simulink model "PMSM_SA88_1Motor"  (R2025a)
settings: Solver=ode4  StartTime=0.0  StopTime=StopTime  FixedStep=Ts_solver  RelTol=1e-3
values from neighbouring files (symbols this model uses):
  Bm = 1e-3    (= 0.001)    [EMRAX348_DQData.m]    (also in Evolito_D500_DQData.m; pmsm_batt_testbench_data.m)
  C1_pack = (Np/Ns)*c1_cell    [pmsm_batt_testbench_data.m]
  Cap_pack = Np*Cell_Cap    (= 700)    [pmsm_batt_testbench_data.m]
  Imax = 1070    [EMRAX348_DQData.m]    (also in Evolito_D500_DQData.m = 1450; pmsm_batt_testbench_data.m = 1450)
  Jtot = 2.0    (= 2)    [pmsm_batt_testbench_data.m]
  Ki_i = Rs*bw_i    (= 18.8495559215)    [pmsm_batt_testbench_data.m]
  Ki_w = Kp_w*bw_w/10    (= 292.432722995)    [pmsm_batt_testbench_data.m]
  Kp_i = Ld*bw_i    (= 0.251327412287)    [pmsm_batt_testbench_data.m]
  Kp_w = Jtot*bw_w/Kt    (= 93.084226773)    [pmsm_batt_testbench_data.m]
  Ld = 52e-6    (= 5.2e-05)    [EMRAX348_DQData.m]    (also in Evolito_D500_DQData.m = 4e-05; pmsm_batt_testbench_data.m = 4e-05)
  Lq = 52e-6    (= 5.2e-05)    [EMRAX348_DQData.m]    (also in Evolito_D500_DQData.m = 4e-05; pmsm_batt_testbench_data.m = 4e-05)
  OCV_pack = Ns*ocv_cell    [pmsm_batt_testbench_data.m]
  p = 10    [EMRAX348_DQData.m]    (also in Evolito_D500_DQData.m; pmsm_batt_testbench_data.m)
  psim = 0.06249    [EMRAX348_DQData.m]    (also in Evolito_D500_DQData.m = 0.045; pmsm_batt_testbench_data.m = 0.045)
  R0_pack = (Ns/Np)*rs_cell    [pmsm_batt_testbench_data.m]
  R1_pack = (Ns/Np)*r1_cell    [pmsm_batt_testbench_data.m]
  Rs = 0.00474    [EMRAX348_DQData.m]    (also in Evolito_D500_DQData.m = 0.004; pmsm_batt_testbench_data.m = 0.003)
  SOC0 = 0.90    (= 0.9)    [pmsm_batt_testbench_data.m]
  tau_dc = 1e-4    (= 0.0001)    [pmsm_batt_testbench_data.m]
  w_ref_val = [724.9; 726.5; 725.1; 726.7]    [pmsm_batt_testbench_data.m]
undefined symbols (not defined in the file or in its folder): soc_bp
libraries: slpidlib x3, simulink x1
settings Model: Creator=froshoo  LastModifiedBy=froshoo

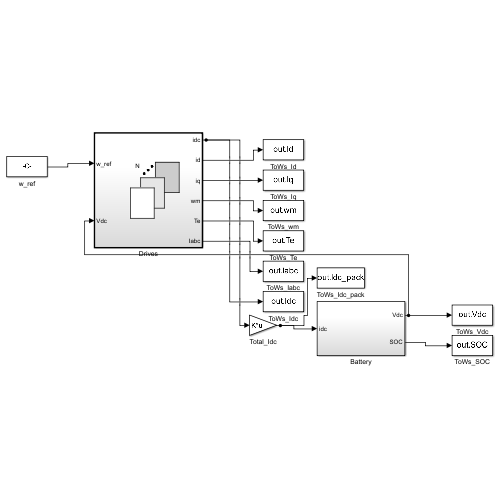
[thumbnail: Simulink's stored preview of the top-level diagram]
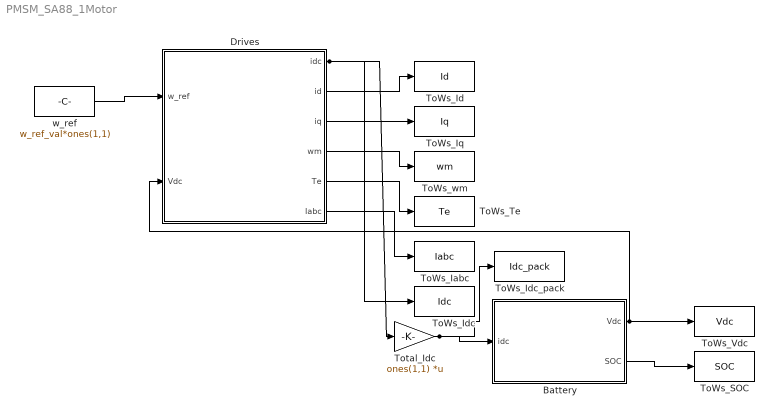
== system PMSM_SA88_1Motor ==
  Battery : Subsystem
  Drives : Subsystem  TreatAsAtomicUnit=on
  ToWs_Iabc : ToWorkspace  VariableName=Iabc  SaveFormat=Timeseries  SampleTime=-1
  ToWs_Id : ToWorkspace  VariableName=Id  SaveFormat=Timeseries  SampleTime=-1
  ToWs_Idc : ToWorkspace  VariableName=Idc  SaveFormat=Timeseries  SampleTime=-1
  ToWs_Idc_pack : ToWorkspace  VariableName=Idc_pack  SaveFormat=Timeseries  SampleTime=-1
  ToWs_Iq : ToWorkspace  VariableName=Iq  SaveFormat=Timeseries  SampleTime=-1
  ToWs_SOC : ToWorkspace  VariableName=SOC  SaveFormat=Timeseries  SampleTime=-1
  ToWs_Te : ToWorkspace  VariableName=Te  SaveFormat=Timeseries  SampleTime=-1
  ToWs_Vdc : ToWorkspace  VariableName=Vdc  SaveFormat=Timeseries  SampleTime=-1
  ToWs_wm : ToWorkspace  VariableName=wm  SaveFormat=Timeseries  SampleTime=-1
  Total_Idc : Gain  Gain=ones(1,1)  Multiplication=Matrix(K*u)
  w_ref : Constant  Value=w_ref_val*ones(1,1)
  wires:
  w_ref/1 -> Drives/1(w_ref)
  Battery/1(Vdc) -> Drives/2(Vdc), ToWs_Vdc/1
  Drives/1(idc) -> Total_Idc/1, ToWs_Idc/1
  Total_Idc/1 -> Battery/1(idc), ToWs_Idc_pack/1
  Drives/2(id) -> ToWs_Id/1
  Drives/3(iq) -> ToWs_Iq/1
  Drives/4(wm) -> ToWs_wm/1
  Drives/5(Te) -> ToWs_Te/1
  Drives/6(Iabc) -> ToWs_Iabc/1
  Battery/2(SOC) -> ToWs_SOC/1

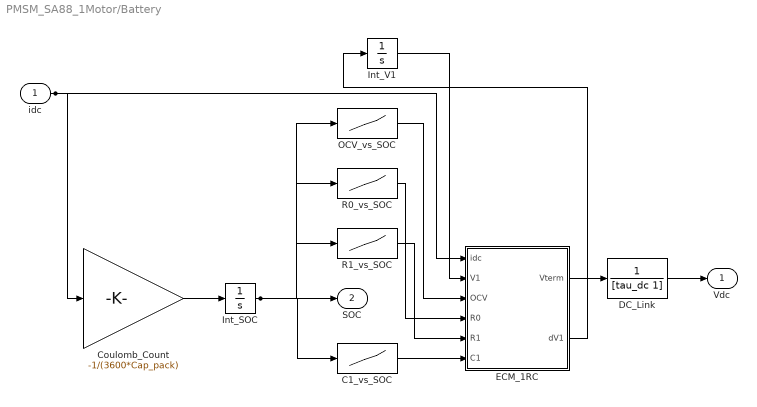
== system PMSM_SA88_1Motor/Battery ==
  idc : Inport
  C1_vs_SOC : Lookup_n-D  NumberOfTableDimensions=1  BreakpointsForDimension1=soc_bp  Table=C1_pack  InternalRulePriority=Speed  RndMeth=Simplest
  Coulomb_Count : Gain  Gain=-1/(3600*Cap_pack)
  DC_Link : TransferFcn  Denominator=[tau_dc 1]
  ECM_1RC : MATLAB Function  TreatAsAtomicUnit=on
  Int_SOC : Integrator  InitialCondition=SOC0
  Int_V1 : Integrator
  OCV_vs_SOC : Lookup_n-D  NumberOfTableDimensions=1  BreakpointsForDimension1=soc_bp  Table=OCV_pack  InternalRulePriority=Speed  RndMeth=Simplest
  R0_vs_SOC : Lookup_n-D  NumberOfTableDimensions=1  BreakpointsForDimension1=soc_bp  Table=R0_pack  InternalRulePriority=Speed  RndMeth=Simplest
  R1_vs_SOC : Lookup_n-D  NumberOfTableDimensions=1  BreakpointsForDimension1=soc_bp  Table=R1_pack  InternalRulePriority=Speed  RndMeth=Simplest
  Vdc : Outport
  SOC : Outport  Port=2
  wires:
  Int_V1/1 -> ECM_1RC/2(V1)
  idc/1 -> ECM_1RC/1(idc), Coulomb_Count/1
  Coulomb_Count/1 -> Int_SOC/1
  R0_vs_SOC/1 -> ECM_1RC/4(R0)
  Int_SOC/1 -> R0_vs_SOC/1, OCV_vs_SOC/1, SOC/1, C1_vs_SOC/1, R1_vs_SOC/1
  OCV_vs_SOC/1 -> ECM_1RC/3(OCV)
  R1_vs_SOC/1 -> ECM_1RC/5(R1)
  C1_vs_SOC/1 -> ECM_1RC/6(C1)
  ECM_1RC/2(dV1) -> Int_V1/1
  ECM_1RC/1(Vterm) -> DC_Link/1
  DC_Link/1 -> Vdc/1

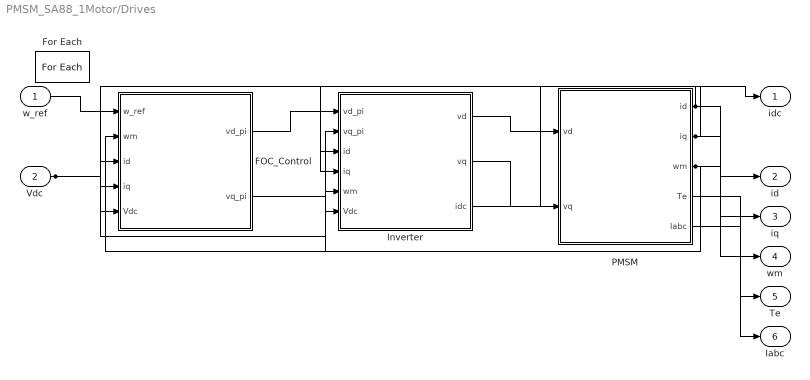
== system PMSM_SA88_1Motor/Drives ==
  w_ref : Inport  Partition=on  PartitionDimension=1  PartitionWidth=1  PartitionOffset=0
  Vdc : Inport  Port=2
  FOC_Control : Subsystem
  For Each : ForEach  DisableCoverage=on  SpecifiedNumIters=1
  Inverter : Subsystem
  PMSM : Subsystem
  idc : Outport  ConcatenationDimension=1
  id : Outport  Port=2  ConcatenationDimension=1
  iq : Outport  Port=3  ConcatenationDimension=1
  wm : Outport  Port=4  ConcatenationDimension=1
  Te : Outport  Port=5  ConcatenationDimension=1
  Iabc : Outport  Port=6  ConcatenationDimension=1
  wires:
  w_ref/1 -> FOC_Control/1(w_ref)
  PMSM/3(wm) -> FOC_Control/2(wm), Inverter/5(wm), wm/1
  PMSM/1(id) -> FOC_Control/3(id), Inverter/3(id), id/1
  PMSM/2(iq) -> FOC_Control/4(iq), Inverter/4(iq), iq/1
  Vdc/1 -> FOC_Control/5(Vdc), Inverter/6(Vdc)
  FOC_Control/1(vd_pi) -> Inverter/1(vd_pi)
  FOC_Control/2(vq_pi) -> Inverter/2(vq_pi)
  Inverter/1(vd) -> PMSM/1(vd)
  Inverter/2(vq) -> PMSM/2(vq)
  Inverter/3(idc) -> idc/1
  PMSM/4(Te) -> Te/1
  PMSM/5(Iabc) -> Iabc/1

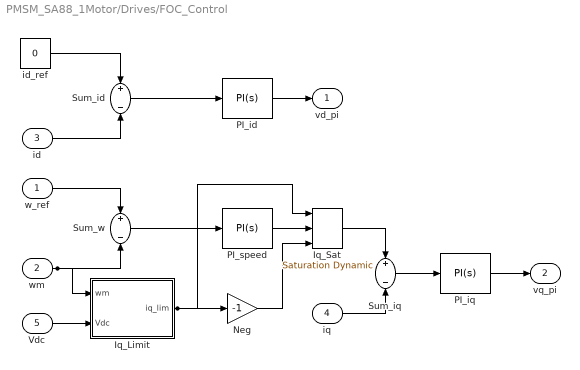
== system PMSM_SA88_1Motor/Drives/FOC_Control ==
  w_ref : Inport
  wm : Inport  Port=2
  id : Inport  Port=3
  iq : Inport  Port=4
  Vdc : Inport  Port=5
  Iq_Limit : MATLAB Function  TreatAsAtomicUnit=on
  Iq_Sat : simulink/Discontinuities/Saturation Dynamic  OutMin=[]  OutMax=[]  OutDataTypeStr=Inherit: Same as second input  OutDataType=fixdt(1, 16)  OutScaling=2^-10  DoSatur=off
  Neg : Gain  Gain=-1
  PI_id : slpidlib/PID Controller  Controller=PI  Form=Parallel  TimeDomain=Continuous-time  UseExternalTs=off  SampleTime=-1  IntegratorMethod=Forward Euler  FilterMethod=Forward Euler  ControllerParametersSource=internal  P=Kp_i  I=Ki_i  UseKiTs=off  D=0  UseExternalDerivativeSource=off  N=100  UseFilter=on  TunerSelectOption=Transfer Function Based (PID Tuner App)  InitialConditionSource=internal  InitialConditionForIntegrator=0  InitialConditionForFilter=0  DifferentiatorICPrevScaledInput=0  ExternalReset=none  TrackingMode=off  Kt=1  LimitOutput=off  SatLimitsSource=internal  UpperSaturationLimit=inf  LowerSaturationLimit=-inf  LinearizeAsGain=on  AntiWindupMode=none  Kb=1  LimitIntegrator=off  UpperIntegratorSaturationLimit=inf  LowerIntegratorSaturationLimit=-inf  POutMin=[]  POutMax=[]  IOutMin=[]  IOutMax=[]  DOutMin=[]  DOutMax=[]  NOutMin=[]  NOutMax=[]  SumOutMin=[]  SumOutMax=[]  SaturationOutMin=[]  SaturationOutMax=[]  PParamMin=[]  PParamMax=[]  IParamMin=[]  IParamMax=[]  DParamMin=[]  DParamMax=[]  NParamMin=[]  NParamMax=[]  KbParamMin=[]  KbParamMax=[]  KtParamMin=[]  KtParamMax=[]  KbOutMin=[]  KbOutMax=[]  KtOutMin=[]  KtOutMax=[]  IntegratorOutMin=[]  IntegratorOutMax=[]  FilterOutMin=[]  FilterOutMax=[]  SumI1OutMin=[]  SumI1OutMax=[]  SumI2OutMin=[]  SumI2OutMax=[]  SumI3OutMin=[]  SumI3OutMax=[]  SumI4OutMin=[]  SumI4OutMax=[]  SumDOutMin=[]  SumDOutMax=[]  DifferentiatorOutMin=[]  DifferentiatorOutMax=[]  FilterDiffOutCoefMin=[]  FilterDiffOutCoefMax=[]  ReciprocalOutMin=[]  ReciprocalOutMax=[]  SumDenOutMin=[]  SumDenOutMax=[]  SumNumOutMin=[]  SumNumOutMax=[]  DivideOutMin=[]  DivideOutMax=[]  UdiffTsProdOutMin=[]  UdiffTsProdOutMax=[]  NTsProdOutMin=[]  NTsProdOutMax=[]  UintegralTsProdOutMin=[]  UintegralTsProdOutMax=[]  UngainTsProdOutMin=[]  UngainTsProdOutMax=[]  ClampingZeroOutDataTypeStr=Inherit: Inherit via back propagation  ClampingZeroOutMin=[]  ClampingZeroOutMax=[]  FilterDenConstantOutDataTypeStr=Inherit: Inherit via back propagation  FilterDenConstantOutMin=[]  FilterDenConstantOutMax=[]  PCopyOutDataTypeStr=Inherit: Inherit via back propagation  PCopyOutMin=[]  PCopyOutMax=[]  NCopyOutDataTypeStr=Inherit: Inherit via back propagation  NCopyOutMin=[]  NCopyOutMax=[]  IntegratorContinuousStateAttributes=''  IntegratorStateMustResolveToSignalObject=off  IntegratorRTWStateStorageClass=Auto  FilterContinuousStateAttributes=''  FilterStateMustResolveToSignalObject=off  FilterRTWStateStorageClass=Auto  ParallelPVariant=InternalParameters  IdealPVariant=Disabled  IVariant=InternalParameters  DVariant=Disabled  IntegratorVariant=Continuous  SatVariant=Disabled  AWVariant=Passthrough  PCopyVariant=Disabled  TRVariant=Disabled  FdbkBlocksVariant=Forward  IdealPFdbkVariant=Disabled  SatFdbkVariant=Disabled  DerivativeFilterVariant=Disabled  NVariant=Disabled  NCopyVariant=Disabled_SignalSpec  FilterICVariant=Disabled  IntegratorICVariant=InternalICs  ExternalResetVariant=Disabled  TRSumVariant=Passthrough  SumFdbkVariant=Disabled  SumVariant=Sum_PI  TsampFilterVariant=InternalTs  TsampNgainVariant=Passthrough  TsampIntegralVariant=Disabled_SignalSpec  ExternalSaturationOutDataTypeStr=Inherit: Same as second input  DerivativeSourceVariant=Disabled  PreIntVariant=InternalPreInt
  PI_iq : slpidlib/PID Controller  Controller=PI  Form=Parallel  TimeDomain=Continuous-time  UseExternalTs=off  SampleTime=-1  IntegratorMethod=Forward Euler  FilterMethod=Forward Euler  ControllerParametersSource=internal  P=Kp_i  I=Ki_i  UseKiTs=off  D=0  UseExternalDerivativeSource=off  N=100  UseFilter=on  TunerSelectOption=Transfer Function Based (PID Tuner App)  InitialConditionSource=internal  InitialConditionForIntegrator=0  InitialConditionForFilter=0  DifferentiatorICPrevScaledInput=0  ExternalReset=none  TrackingMode=off  Kt=1  LimitOutput=off  SatLimitsSource=internal  UpperSaturationLimit=inf  LowerSaturationLimit=-inf  LinearizeAsGain=on  AntiWindupMode=none  Kb=1  LimitIntegrator=off  UpperIntegratorSaturationLimit=inf  LowerIntegratorSaturationLimit=-inf  POutMin=[]  POutMax=[]  IOutMin=[]  IOutMax=[]  DOutMin=[]  DOutMax=[]  NOutMin=[]  NOutMax=[]  SumOutMin=[]  SumOutMax=[]  SaturationOutMin=[]  SaturationOutMax=[]  PParamMin=[]  PParamMax=[]  IParamMin=[]  IParamMax=[]  DParamMin=[]  DParamMax=[]  NParamMin=[]  NParamMax=[]  KbParamMin=[]  KbParamMax=[]  KtParamMin=[]  KtParamMax=[]  KbOutMin=[]  KbOutMax=[]  KtOutMin=[]  KtOutMax=[]  IntegratorOutMin=[]  IntegratorOutMax=[]  FilterOutMin=[]  FilterOutMax=[]  SumI1OutMin=[]  SumI1OutMax=[]  SumI2OutMin=[]  SumI2OutMax=[]  SumI3OutMin=[]  SumI3OutMax=[]  SumI4OutMin=[]  SumI4OutMax=[]  SumDOutMin=[]  SumDOutMax=[]  DifferentiatorOutMin=[]  DifferentiatorOutMax=[]  FilterDiffOutCoefMin=[]  FilterDiffOutCoefMax=[]  ReciprocalOutMin=[]  ReciprocalOutMax=[]  SumDenOutMin=[]  SumDenOutMax=[]  SumNumOutMin=[]  SumNumOutMax=[]  DivideOutMin=[]  DivideOutMax=[]  UdiffTsProdOutMin=[]  UdiffTsProdOutMax=[]  NTsProdOutMin=[]  NTsProdOutMax=[]  UintegralTsProdOutMin=[]  UintegralTsProdOutMax=[]  UngainTsProdOutMin=[]  UngainTsProdOutMax=[]  ClampingZeroOutDataTypeStr=Inherit: Inherit via back propagation  ClampingZeroOutMin=[]  ClampingZeroOutMax=[]  FilterDenConstantOutDataTypeStr=Inherit: Inherit via back propagation  FilterDenConstantOutMin=[]  FilterDenConstantOutMax=[]  PCopyOutDataTypeStr=Inherit: Inherit via back propagation  PCopyOutMin=[]  PCopyOutMax=[]  NCopyOutDataTypeStr=Inherit: Inherit via back propagation  NCopyOutMin=[]  NCopyOutMax=[]  IntegratorContinuousStateAttributes=''  IntegratorStateMustResolveToSignalObject=off  IntegratorRTWStateStorageClass=Auto  FilterContinuousStateAttributes=''  FilterStateMustResolveToSignalObject=off  FilterRTWStateStorageClass=Auto  ParallelPVariant=InternalParameters  IdealPVariant=Disabled  IVariant=InternalParameters  DVariant=Disabled  IntegratorVariant=Continuous  SatVariant=Disabled  AWVariant=Passthrough  PCopyVariant=Disabled  TRVariant=Disabled  FdbkBlocksVariant=Forward  IdealPFdbkVariant=Disabled  SatFdbkVariant=Disabled  DerivativeFilterVariant=Disabled  NVariant=Disabled  NCopyVariant=Disabled_SignalSpec  FilterICVariant=Disabled  IntegratorICVariant=InternalICs  ExternalResetVariant=Disabled  TRSumVariant=Passthrough  SumFdbkVariant=Disabled  SumVariant=Sum_PI  TsampFilterVariant=InternalTs  TsampNgainVariant=Passthrough  TsampIntegralVariant=Disabled_SignalSpec  ExternalSaturationOutDataTypeStr=Inherit: Same as second input  DerivativeSourceVariant=Disabled  PreIntVariant=InternalPreInt
  PI_speed : slpidlib/PID Controller  Controller=PI  Form=Parallel  TimeDomain=Continuous-time  UseExternalTs=off  SampleTime=-1  IntegratorMethod=Forward Euler  FilterMethod=Forward Euler  ControllerParametersSource=internal  P=Kp_w  I=Ki_w  UseKiTs=off  D=0  UseExternalDerivativeSource=off  N=100  UseFilter=on  TunerSelectOption=Transfer Function Based (PID Tuner App)  InitialConditionSource=internal  InitialConditionForIntegrator=0  InitialConditionForFilter=0  DifferentiatorICPrevScaledInput=0  ExternalReset=none  TrackingMode=off  Kt=1  LimitOutput=on  SatLimitsSource=internal  UpperSaturationLimit=Imax  LowerSaturationLimit=-Imax  LinearizeAsGain=on  AntiWindupMode=back-calculation  Kb=1  LimitIntegrator=off  UpperIntegratorSaturationLimit=inf  LowerIntegratorSaturationLimit=-inf  POutMin=[]  POutMax=[]  IOutMin=[]  IOutMax=[]  DOutMin=[]  DOutMax=[]  NOutMin=[]  NOutMax=[]  SumOutMin=[]  SumOutMax=[]  SaturationOutMin=[]  SaturationOutMax=[]  PParamMin=[]  PParamMax=[]  IParamMin=[]  IParamMax=[]  DParamMin=[]  DParamMax=[]  NParamMin=[]  NParamMax=[]  KbParamMin=[]  KbParamMax=[]  KtParamMin=[]  KtParamMax=[]  KbOutMin=[]  KbOutMax=[]  KtOutMin=[]  KtOutMax=[]  IntegratorOutMin=[]  IntegratorOutMax=[]  FilterOutMin=[]  FilterOutMax=[]  SumI1OutMin=[]  SumI1OutMax=[]  SumI2OutMin=[]  SumI2OutMax=[]  SumI3OutMin=[]  SumI3OutMax=[]  SumI4OutMin=[]  SumI4OutMax=[]  SumDOutMin=[]  SumDOutMax=[]  DifferentiatorOutMin=[]  DifferentiatorOutMax=[]  FilterDiffOutCoefMin=[]  FilterDiffOutCoefMax=[]  ReciprocalOutMin=[]  ReciprocalOutMax=[]  SumDenOutMin=[]  SumDenOutMax=[]  SumNumOutMin=[]  SumNumOutMax=[]  DivideOutMin=[]  DivideOutMax=[]  UdiffTsProdOutMin=[]  UdiffTsProdOutMax=[]  NTsProdOutMin=[]  NTsProdOutMax=[]  UintegralTsProdOutMin=[]  UintegralTsProdOutMax=[]  UngainTsProdOutMin=[]  UngainTsProdOutMax=[]  ClampingZeroOutDataTypeStr=Inherit: Inherit via back propagation  ClampingZeroOutMin=[]  ClampingZeroOutMax=[]  FilterDenConstantOutDataTypeStr=Inherit: Inherit via back propagation  FilterDenConstantOutMin=[]  FilterDenConstantOutMax=[]  PCopyOutDataTypeStr=Inherit: Inherit via back propagation  PCopyOutMin=[]  PCopyOutMax=[]  NCopyOutDataTypeStr=Inherit: Inherit via back propagation  NCopyOutMin=[]  NCopyOutMax=[]  IntegratorContinuousStateAttributes=''  IntegratorStateMustResolveToSignalObject=off  IntegratorRTWStateStorageClass=Auto  FilterContinuousStateAttributes=''  FilterStateMustResolveToSignalObject=off  FilterRTWStateStorageClass=Auto  ParallelPVariant=InternalParameters  IdealPVariant=Disabled  IVariant=InternalParameters  DVariant=Disabled  IntegratorVariant=Continuous  SatVariant=Enabled  AWVariant=BackCalculation  PCopyVariant=Disabled  TRVariant=Disabled  FdbkBlocksVariant=Forward  IdealPFdbkVariant=Disabled  SatFdbkVariant=Disabled  DerivativeFilterVariant=Disabled  NVariant=Disabled  NCopyVariant=Disabled_SignalSpec  FilterICVariant=Disabled  IntegratorICVariant=InternalICs  ExternalResetVariant=Disabled  TRSumVariant=Passthrough  SumFdbkVariant=Disabled  SumVariant=Sum_PI  TsampFilterVariant=InternalTs  TsampNgainVariant=Passthrough  TsampIntegralVariant=Disabled_SignalSpec  ExternalSaturationOutDataTypeStr=Inherit: Same as second input  DerivativeSourceVariant=Disabled  PreIntVariant=InternalPreInt
  Sum_id : Sum  Inputs=+-
  Sum_iq : Sum  Inputs=+-
  Sum_w : Sum  Inputs=+-
  id_ref : Constant  Value=0
  vd_pi : Outport
  vq_pi : Outport  Port=2
  wires:
  Vdc/1 -> Iq_Limit/2(Vdc)
  id_ref/1 -> Sum_id/1
  wm/1 -> Sum_w/2, Iq_Limit/1(wm)
  PI_iq/1 -> vq_pi/1
  w_ref/1 -> Sum_w/1
  id/1 -> Sum_id/2
  Sum_iq/1 -> PI_iq/1
  Sum_id/1 -> PI_id/1
  Sum_w/1 -> PI_speed/1
  Iq_Limit/1(iq_lim) -> Iq_Sat/1, Neg/1
  PI_id/1 -> vd_pi/1
  PI_speed/1 -> Iq_Sat/2
  Neg/1 -> Iq_Sat/3
  Iq_Sat/1 -> Sum_iq/1
  iq/1 -> Sum_iq/2

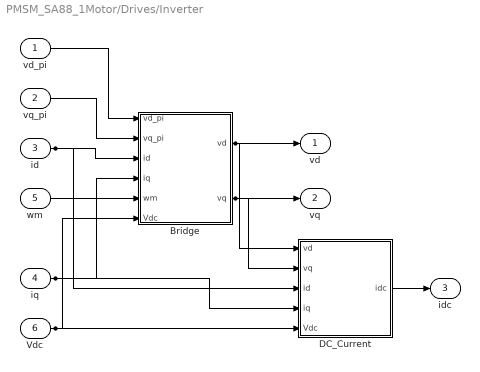
== system PMSM_SA88_1Motor/Drives/Inverter ==
  vd_pi : Inport
  vq_pi : Inport  Port=2
  id : Inport  Port=3
  iq : Inport  Port=4
  wm : Inport  Port=5
  Vdc : Inport  Port=6
  Bridge : MATLAB Function  TreatAsAtomicUnit=on
  DC_Current : MATLAB Function  TreatAsAtomicUnit=on
  vd : Outport
  vq : Outport  Port=2
  idc : Outport  Port=3
  wires:
  vd_pi/1 -> Bridge/1(vd_pi)
  vq_pi/1 -> Bridge/2(vq_pi)
  Vdc/1 -> DC_Current/5(Vdc), Bridge/6(Vdc)
  id/1 -> DC_Current/3(id), Bridge/3(id)
  Bridge/1(vd) -> vd/1, DC_Current/1(vd)
  wm/1 -> Bridge/5(wm)
  Bridge/2(vq) -> vq/1, DC_Current/2(vq)
  iq/1 -> Bridge/4(iq), DC_Current/4(iq)
  DC_Current/1(idc) -> idc/1

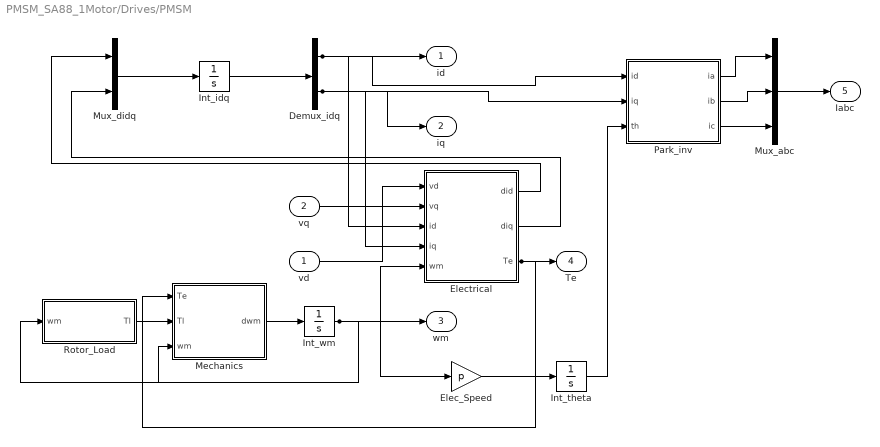
== system PMSM_SA88_1Motor/Drives/PMSM ==
  vd : Inport
  vq : Inport  Port=2
  Demux_idq : Demux  Outputs=2
  Elec_Speed : Gain  Gain=p
  Electrical : MATLAB Function  TreatAsAtomicUnit=on
  Int_idq : Integrator  InitialCondition=[0;0]
  Int_theta : Integrator
  Int_wm : Integrator
  Mechanics : MATLAB Function  TreatAsAtomicUnit=on
  Mux_abc : Mux  Inputs=3
  Mux_didq : Mux  Inputs=2
  Park_inv : MATLAB Function  TreatAsAtomicUnit=on
  Rotor_Load : MATLAB Function  TreatAsAtomicUnit=on
  id : Outport
  iq : Outport  Port=2
  wm : Outport  Port=3
  Te : Outport  Port=4
  Iabc : Outport  Port=5
  wires:
  Mux_didq/1 -> Int_idq/1
  Demux_idq/2 -> Park_inv/2(iq), Electrical/4(iq), iq/1
  Rotor_Load/1(Tl) -> Mechanics/2(Tl)
  Mux_abc/1 -> Iabc/1
  Park_inv/2(ib) -> Mux_abc/2
  vd/1 -> Electrical/1(vd)
  Int_idq/1 -> Demux_idq/1
  Mechanics/1(dwm) -> Int_wm/1
  Demux_idq/1 -> Park_inv/1(id), Electrical/3(id), id/1
  vq/1 -> Electrical/2(vq)
  Int_wm/1 -> Rotor_Load/1(wm), Electrical/5(wm), wm/1, Mechanics/3(wm), Elec_Speed/1
  Electrical/3(Te) -> Mechanics/1(Te), Te/1
  Electrical/1(did) -> Mux_didq/1
  Electrical/2(diq) -> Mux_didq/2
  Elec_Speed/1 -> Int_theta/1
  Int_theta/1 -> Park_inv/3(th)
  Park_inv/1(ia) -> Mux_abc/1
  Park_inv/3(ic) -> Mux_abc/3

== matlab function PMSM_SA88_1Motor/Battery/ECM_1RC ==
  data: idc input size=1; Vterm output size=1; V1 input size=1; OCV input size=1; R0 input size=1; R1 input size=1; C1 input size=1; dV1 output size=1
function [Vterm, dV1] = fcn(idc, V1, OCV, R0, R1, C1)
%#codegen
% SA88 pack, 1-RC equivalent-circuit model. idc is the TOTAL pack current
% (all motors summed). Discharge (idc > 0) pulls the terminal voltage below
% the open-circuit voltage -- this is what couples the motors to each other.
%   Vterm = OCV(SOC) - idc*R0(SOC) - V1
%   dV1/dt = idc/C1 - V1/(R1*C1)
Vterm = OCV - idc*R0 - V1;
dV1   = idc/C1 - V1/(R1*C1);

== matlab function PMSM_SA88_1Motor/Drives/Inverter/Bridge ==
  data: vd_pi input size=1; vd output size=1; vq_pi input size=1; id input size=1; iq input size=1; wm input size=1; Vdc input size=1; vq output size=1; p parameter; Ld parameter; Lq parameter; psim parameter
function [vd, vq] = fcn(vd_pi, vq_pi, id, iq, wm, Vdc, p, Ld, Lq, psim)
%#codegen
% Averaged inverter: no switching, so no PWM ripple -- the dq voltage command
% is applied directly. Two things happen here:
%  1) dq decoupling feedforward. The PI outputs only have to cover the
%     resistive drop and transients; the back-EMF and the we*L cross-coupling
%     are cancelled. Without this the d-axis loses control near the voltage
%     limit and id drifts positive (which raises the flux and makes it worse).
%  2) clamp onto the SVPWM linear-range circle, Vmax = Vdc/sqrt(3).
we   = p*wm;
vd_c = vd_pi - we*Lq*iq;
vq_c = vq_pi + we*(Ld*id + psim);
Vmax = Vdc/sqrt(3);
Vm   = sqrt(vd_c^2 + vq_c^2);
if Vm > Vmax && Vm > 0
    k = Vmax/Vm;
else
    k = 1;
end
vd = k*vd_c;
vq = k*vq_c;

== matlab function PMSM_SA88_1Motor/Drives/FOC_Control/Iq_Limit ==
  data: wm input size=1; iq_lim output size=1; Vdc input size=1; p parameter; psim parameter; Lq parameter; Imax parameter
function iq_lim = fcn(wm, Vdc, p, psim, Lq, Imax)
%#codegen
% Largest iq the bus can actually drive at this speed (with id = 0):
%   (we*psim + Rs*iq)^2 + (we*Lq*iq)^2 <= Vmax^2
% Dropping the small Rs*iq term -> iq <= sqrt(Vmax^2-(we*psim)^2)/(we*Lq).
% A flat Imax limit would command an iq the bus cannot support, the inverter
% would saturate and the current PIs would wind up (id runs away).
we   = p*abs(wm);
Vmax = Vdc/sqrt(3);
Eb   = we*psim;
marg = Vmax^2 - Eb^2;
if we < 1 || marg <= 0
    iq_v = Imax;
else
    iq_v = sqrt(marg)/(we*Lq);
end
iq_lim = min(Imax, iq_v);

== matlab function PMSM_SA88_1Motor/Drives/Inverter/DC_Current ==
  data: vd input size=1; idc output size=1; vq input size=1; id input size=1; iq input size=1; Vdc input size=1
function idc = fcn(vd, vq, id, iq, Vdc)
%#codegen
% DC-side current from AC power balance (averaged inverter, lossless).
% This is what ties the AC side to the battery: Pdc = Pac.
Pac = 1.5*(vd*id + vq*iq);
idc = Pac/max(Vdc, 1);

== matlab function PMSM_SA88_1Motor/Drives/PMSM/Electrical ==
  data: vd input size=1; did output size=1; vq input size=1; id input size=1; iq input size=1; wm input size=1; diq output size=1; Te output size=1; p parameter; Rs parameter; Ld parameter; Lq parameter; psim parameter
function [did, diq, Te] = fcn(vd, vq, id, iq, wm, p, Rs, Ld, Lq, psim)
%#codegen
% PMSM stator equations in the rotor dq frame. This block is deliberately
% stateless: it returns the DERIVATIVES and the Integrator blocks outside own
% the states, so ode4 integrates them properly (a persistent variable here
% would silently degrade the motor states to forward Euler).
we  = p*wm;
did = (vd - Rs*id + we*Lq*iq)/Ld;
diq = (vq - Rs*iq - we*(Ld*id + psim))/Lq;
% With Ld = Lq (non-salient) the reluctance term vanishes and Te = 1.5*p*psim*iq.
Te  = 1.5*p*(psim*iq + (Ld - Lq)*id*iq);

== matlab function PMSM_SA88_1Motor/Drives/PMSM/Rotor_Load ==
  data: wm input size=1; Tl output size=1; k_drag parameter
function Tl = fcn(wm, k_drag)
%#codegen
% Rotor aerodynamic drag torque, calibrated from the P4 flight run:
% hover at 724.9 rad/s draws 668 N*m. A least-squares fit of Tq vs w^2 over
% the whole mission gives the same k_drag, so the w^2 law holds well.
Tl = k_drag*wm*abs(wm);

== matlab function PMSM_SA88_1Motor/Drives/PMSM/Mechanics ==
  data: Te input size=1; dwm output size=1; Tl input size=1; wm input size=1; Bm parameter; Jtot parameter
function dwm = fcn(Te, Tl, wm, Bm, Jtot)
%#codegen
dwm = (Te - Tl - Bm*wm)/Jtot;

== matlab function PMSM_SA88_1Motor/Drives/PMSM/Park_inv ==
  data: id input size=1; ia output size=1; iq input size=1; th input size=1; ib output size=1; ic output size=1
function [ia, ib, ic] = fcn(id, iq, th)
%#codegen
% inverse Park + inverse Clarke (amplitude-invariant): dq -> abc.
% The fast oscillation comes from th = integral(p*wm); the amplitude is iq.
ia = id*cos(th)        - iq*sin(th);
ib = id*cos(th-2*pi/3) - iq*sin(th-2*pi/3);
ic = id*cos(th+2*pi/3) - iq*sin(th+2*pi/3);
